simulink model "l512_devel_pps_2016f"  (R2012b)
settings: Solver=ode45  StartTime=0.0  StopTime=15000  RelTol=1e-3
undefined symbols (not defined in the file): sfp
libraries: xbsIndex_r4 x7383, casper_library_misc x259, casper_library_delays x118, xps_library x12, simulink x1
(part 1 of 82)
settings Model: ModifiedComment=dprice -- Thu Mar 24 21:54:32 2016 -- Version 1.495  Creator=jkocz  LastModifiedBy=dprice
settings Model: ModifiedHistory=|
  | dprice -- Thu Mar 24 21:54:32 2016 -- Version 1.495
  | 
  | 
  | dprice -- Thu Mar 24 13:03:20 2016 -- Version 1.494
  | Made by own dual_pol delay block :/
  | SCREW YOU WIDEBAND_PROG YOU PIECE OF SHIT
  | 
  | dprice -- Thu Mar 24 12:42:23 2016 -- Version 1.493
  | About to change coarse delay so it's not a pile of shit
  | 
  | dprice -- Wed Mar 16 15:57:57 2016 -- Version 1.492
  | 
  | 
  | dprice -- Mon Feb 22 14:48:29 2016 -- Version 1.491
  | updated to 2048 max delay
  | 
  | dprice -- Mon Feb 01 14:04:02 2016 -- Version 1.490
  | 
  | Added pipeline delays after eq blocks
  | 
  | dprice -- Fri Jan 29 13:04:51 2016 -- Version 1.489
  | 
  | Added pipeline delays on pfb_fir as the timing logs showed this as an issue
  | 
  | dprice -- Wed Jan 27 14:02:19 2016 -- Version 1.488
  | 
  | Changed FFT core
  | 
  | dprice -- Wed Jan 27 13:22:12 2016 -- Version 1.487
  | 
  | Using latest casper_astro_devel more recent FFT
  | 
  | dprice -- Fri Jan 22 10:59:16 2016 -- Version 1.486
  | Added in old tenge core
  | 
  | dprice -- Fri Jan 22 10:26:56 2016 -- Version 1.485
  | about to change tengbe block out
  | 
  | dprice -- Thu Jan 21 17:16:55 2016 -- Version 1.484
  | 
  | 
  | dprice -- Wed Jan 20 11:44:21 2016 -- Version 1.483
  | 
  | Added pipelines around requant mux to help timing
  | 
  | dprice -- Tue Jan 19 16:58:53 2016 -- Version 1.482
  | 
  | 
  | dprice -- Tue Jan 19 16:57:42 2016 -- Version 1.481
  | 
  | added in coarse delay after ADC
  | 
  | dprice -- Tue Jan 19 16:48:56 2016 -- Version 1.480
  | 
  | 
  | dprice -- Tue Jan 19 16:38:05 2016 -- Version 1.479
  | 
  | 
  | dprice -- Tue Jan 19 16:27:23 2016 -- Version 1.478
  | Adding coarse delay
  | 
  | dprice -- Tue Jan 19 15:47:20 2016 -- Version 1.477
  | 
  | 
  | dprice -- Tue Jan 19 15:44:29 2016 -- Version 1.476
  | 
  | 
  | dprice -- Thu Jan 07 01:25:30 2016 -- Version 1.475
  | 
  | Removed goddam FFT preshift shift
  | 
  | dprice -- Mon Jan 04 15:23:51 2016 -- Version 1.474
  | 
  | changed acc_cnt to run up to 2^25 = 1 year
  | 
  | dprice -- Mon Dec 28 14:47:04 2015 -- Version 1.473
  | 
  | Changed requant mux yet again, now can choose in 2 bit steps, from LSB up to -4 from MSB. This will clip RFI
  | 
  | dprice -- Tue Dec 22 18:17:34 2015 -- Version 1.472
  | 
  | Now using simplest requant imaginable: 18 bit slice. Changed vacc toa accept 18 bits, output 32 bits. Allows 14 bits of growth = 2^14 cycles = 16384 cycles = OK
  | 
  | dprice -- Tue Dec 22 18:10:53 2015 -- Version 1.471
  | 
  | 
  | dprice -- Tue Dec 22 16:37:14 2015 -- Version 1.470
  | 
  | Changed bitsel once again, -4 increments
  | 
  | dprice -- Sat Dec 19 20:03:40 2015 -- Version 1.469
  | 
  | Now slicing tops bits only -- can choose 0 - 4 bit offset (12 dB dynamic range). This is more than the sky changes, so should be OK?
  | 
  | dprice -- Thu Dec 17 17:05:01 2015 -- Version 1.468
  | 
  | Changed spectrometer quantization rq
  | 
  | dprice -- Tue Dec 15 08:55:34 2015 -- Version 1.467
  | 
  | Added pipeline delays in tenge block - may have broken something...
  | 
  | dprice -- Tue Dec 15 00:02:55 2015 -- Version 1.466
  | 
  | added dealys before rq mux to help timing. hopefully it compiles now.
  | 
  | dprice -- Mon Dec 14 21:02:26 2015 -- Version 1.465
  | 
  | adding delays back in to see if timing affected. I probably screwed up EOF by just removing it anyways.
  | 
  | dprice -- Mon Dec 14 21:01:23 2015 -- Version 1.464
  | 
  | adding pipeline delay
  | 
  | dprice -- Mon Dec 14 17:37:49 2015 -- Version 1.463
  | 
  | changed spectrometer requeant to do 18_17 -> 16_15.
  | 
  | Removed some random delays in the tenge to see what happens
  | 
  | dprice -- Mon Dec 14 17:35:29 2015 -- Version 1.462
  | 
  | 
  | dprice -- Tue Dec 08 15:27:01 2015 -- Version 1.461
  | 
  | changed requant to just slice the bits of interest
  | 
  | dprice -- Tue Dec 08 15:08:55 2015 -- Version 1.460
  | 
  | Added fft preshift, and fixed bit offset in rq
  | 
  | dprice -- Mon Apr 06 20:09:48 2015 -- Version 1.459
  | Compiled successfully
  | 
  | dprice -- Mon Apr 06 16:18:15 2015 -- Version 1.458
  | 
  | Changed pps delay to about 0.1s
  | 
  | dprice -- Fri Mar 13 15:46:33 2015 -- Version 1.457
  | 
  | 
  | dprice -- Fri Mar 13 15:34:50 2015 -- Version 1.456
  | Copied triggering over to f1 - f4
  | 
  | dprice -- Fri Mar 13 15:31:03 2015 -- Version 1.455
  | 
  | Added better triggering of RMS monitor
  | 
  | dprice -- Wed Jan 21 17:17:07 2015 -- Version 1.454
  | 
  | 
  | dprice -- Wed Jan 21 14:02:39 2015 -- Version 1.453
  | changed to be triggered by correct pps
  | 
  | dprice -- Thu Jan 15 16:51:06 2015 -- Version 1.452
  | dropped core back to 200 MHz from 216 MHz
  | 
  | dprice -- Thu Jan 15 13:30:59 2015 -- Version 1.451
  | 
  | Changed to use PPS triggered vacc. Needs testing!
  | 
  | dprice -- Thu Jan 15 13:21:59 2015 -- Version 1.450
  | 
  | 
  | dprice -- Thu Jan 15 13:19:39 2015 -- Version 1.449
  | 
  | 
  | dprice -- Thu Jan 15 13:13:52 2015 -- Version 1.448
  | 
  | Adding pps triggered vacc
  | 
  | dprice -- Tue Jan 13 15:35:09 2015 -- Version 1.447
  | 
  | Updated to spectrometer f_engine core
  | 
  | dprice -- Wed Dec 17 17:14:12 2014 -- Version 1.446
  | 
  | added some snap blocks to do eq0 output rms tests
  | 
  | dprice -- Fri Nov 21 18:19:20 2014 -- Version 1.445
  | 
  | 
  | dprice -- Fri Nov 21 15:29:28 2014 -- Version 1.444
  | 
  | 
  | dprice -- Fri Nov 21 15:28:21 2014 -- Version 1.443
  | 
  | 
  | dprice -- Fri Nov 21 15:22:12 2014 -- Version 1.442
  | 
  | About to try a compile
  | 
  | dprice -- Fri Nov 21 15:19:27 2014 -- Version 1.441
  | 
  | 
  | dprice -- Fri Nov 21 15:10:28 2014 -- Version 1.440
  | 
  | about to crash :/
  | 
  | dprice -- Thu Dec 19 14:05:55 2013 -- Version 1.439
  | 
  | Removed scope blocks in 10GbE spacketizer
  | 
  | dprice -- Thu Dec 12 01:39:04 2013 -- Version 1.438
  | 
  | Moved pfb and eq to black boxes. Hopefully compile times are a little quicker now...
  | 
  | dprice -- Wed Dec 11 11:19:03 2013 -- Version 1.437
  | 
  | Updated coeff generator (cg) with separate sky BRAM for switching (sw_sky), renamed sky to bpass, and changed from 18 bit to 32 bit coefficients
  | 
  | dprice -- Tue Dec 10 14:55:05 2013 -- Version 1.436
  | 
  | Closing session
  | 
  | dprice -- Sat Dec 07 16:46:59 2013 -- Version 1.435
  | Fixed bool slicing on tgbe_en
  | 
  | dprice -- Wed Dec 04 22:02:25 2013 -- Version 1.434
  | 
  | Trying to compile with 4x gbes in the design
  | 
  | dprice -- Wed Dec 04 21:44:55 2013 -- Version 1.433
  | 
  | Added extra tgbe blocks for failover
  | 
  | dprice -- Wed Dec 04 17:45:31 2013 -- Version 1.432
  | 
  | Renamed coeff_gen cg to save on length of bram name
  | 
  | dprice -- Wed Dec 04 17:38:25 2013 -- Version 1.431
  | 
  | Copied logic across to all fft/fX blocks. Trying first compile.
  | 
  | dprice -- Wed Dec 04 17:29:39 2013 -- Version 1.430
  | 
  | Modified eq block to allow selecting between switched and all-sky modes
  | 
  | dprice -- Wed Dec 04 16:56:15 2013 -- Version 1.429
  | 
  | Adding switching assembly coefficient selection by pps
  | 
  | dprice -- Wed Nov 06 11:09:49 2013 -- Version 1.428
  | 
  | Changed back down to 216 MHz. Added a post-eq snap block for testing of equalization levels
  | 
  | dprice -- Tue Nov 05 18:21:00 2013 -- Version 1.427
  | 
  | Removed scopes as they bring up an irritating message each time you try and compile
  | 
  | dprice -- Tue Nov 05 14:30:34 2013 -- Version 1.426
  | 
  | Found timing issues with round block. Added a mask and increased latency in convert and multiply.
  | 
  | dprice -- Tue Nov 05 11:43:26 2013 -- Version 1.423
  | 
  | Changed clock to 239 MHz, just to see if it still compiles...
  | 
  | dprice -- Tue Nov 05 11:43:26 2013 -- Version 1.423
  | 
  | Changed clock to 239 MHz, just to see if it still compiles...
  | 
  | dprice -- Tue Nov 05 09:11:40 2013 -- Version 1.422
  | 
  | Design compiled successfully at 210 MHz using pblock constraints (hstack). Now bumping to 216 MHz.
  | Added status LEDs to design for PPS and TX
  | 
  | dprice -- Mon Nov 04 16:36:08 2013 -- Version 1.421
  | 
  | Added pipeline delays to yelllow block I/O in effort to aid timing. Worst offending net was the rst yellow block, presumably due to fanout.
  | 
  | Also modified the ADC thresholding logic to use a BRAM vector accumulator.
  | 
  | dprice -- Tue Oct 29 13:55:56 2013 -- Version 1.412
  | 
  | Fixed mux error - due to goto tag mismatch
  | 
  | dprice -- Tue Oct 29 13:55:56 2013 -- Version 1.412
  | 
  | Fixed mux error - due to goto tag mismatch
  | 
  | dprice -- Tue Oct 29 11:53:04 2013 -- Version 1.411
  | 
  | WTF is wrong with these mux blocks? Keep getting error on dtype in on muxes in packetbuffer.
  | 
  | dprice -- Mon Oct 28 18:12:23 2013 -- Version 1.410
  | 
  | 
  | dprice -- Mon Oct 28 18:11:25 2013 -- Version 1.409
  | 
  | Need to remove slice on FFT_SHIFTS
  | 
  | * Black boxed FFT
  | * Added ADC overflow logic and snap.
settings DataIOCC: SignalLoggingSaveFormat=ModelDataLogs
settings DebuggingCC: FcnCallInpInsideContextMsg=UseLocalSettings  StrictBusMsg=Warning
settings GRTTargetCC: CombineOutputUpdateFcns=off  GRTInterface=on

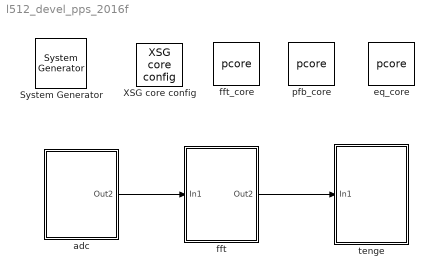
== system l512_devel_pps_2016f ==
  " System Generator" : xbsIndex_r4/ System Generator  Tag=genX  xilinxfamily=virtex6  part=xc6vsx475t  speed=-1  package=ff1759  synthesis_tool=XST  clock_wrapper=Clock Enables  directory=./l512_devel_pps_2016f/sysgen  proj_type=Project Navigator  Synth_file=XST Defaults  Impl_file=ISE Defaults  testbench=off  simulink_period=1  sysclk_period=5  dcm_input_clock_period=100  incr_netlist=off  trim_vbits=Everywhere in SubSystem  dbl_ovrd=According to Block Masks  core_generation=According to Block Masks  run_coregen=off  deprecated_control=off  eval_field=0  block_type=sysgen
      settings: block_version=11.4
  XSG core config : xps_library/XSG core config  Tag=xps:xsg  hw_sys=ROACH2:sx475t  clk_src=adc0_clk  ROACH_clk_src=adc0_clk  ROACH2_clk_src=adc0_clk  clk_rate=200  sample_period=1  synthesis_tool=XST
  adc : Subsystem
  eq_core : xps_library/pcore  Tag=xps:pcore  pcore_path=/data1/dprice/leda512/bb/eq_basic_core/eq_basic_core.ngc
  fft : Subsystem
  fft_core : xps_library/pcore  Tag=xps:pcore  pcore_path=/data1/dprice/leda512/bb/fft_astro_devel_core/fft_astro_devel_core.ngc
  pfb_core : xps_library/pcore  Tag=xps:pcore  pcore_path=/data1/dprice/leda512/bb/pfb_core/pfb_core.ngc
  tenge : Subsystem
  wires:
  adc/1(Out2) -> fft/1(In1)
  fft/1(Out2) -> tenge/1(In1)
